simulink subsystem "global_to_local_waypoint_junho"  (R2022b)
settings: Solver=VariableStepAuto  StartTime=0.0  StopTime=10.0  RelTol=1e-3
libraries: CarMaker4SL x3
settings Model: Creator=USER  LastModifiedBy=USER

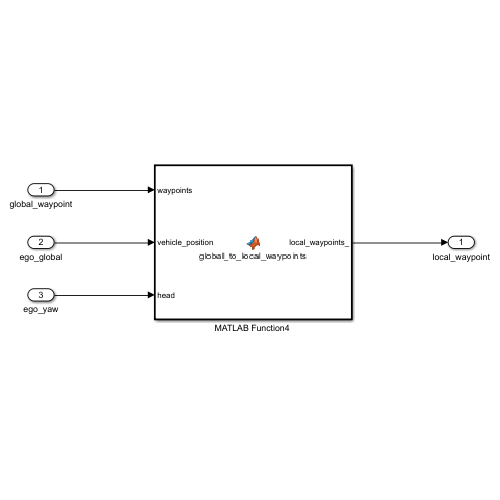
[thumbnail: Simulink's stored preview of the top-level diagram]
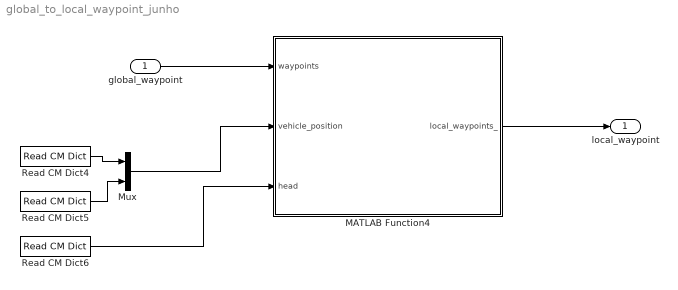
== system global_to_local_waypoint_junho ==
  global_waypoint : Inport
  "MATLAB Function4 " : MATLAB Function  TreatAsAtomicUnit=on
  Mux : Mux  Inputs=2
  Read CM Dict4 : CarMaker4SL/Read CM Dict  xname=Car.Fr1.tx  xsync=off  xstime=Inherited
  Read CM Dict5 : CarMaker4SL/Read CM Dict  xname=Car.Fr1.ty  xsync=off  xstime=Inherited
  Read CM Dict6 : CarMaker4SL/Read CM Dict  xname=Car.Fr1.rz  xsync=off  xstime=Inherited
  local_waypoint : Outport
  wires:
  "MATLAB Function4 "/1(local_waypoints_) -> local_waypoint/1
  global_waypoint/1 -> "MATLAB Function4 "/1(waypoints)
  Read CM Dict4/1 -> Mux/1
  Read CM Dict5/1 -> Mux/2
  Mux/1 -> "MATLAB Function4 "/2(vehicle_position)
  Read CM Dict6/1 -> "MATLAB Function4 "/3(head)

== matlab function global_to_local_waypoint_junho/MATLAB Function4  ==
  settings: updateMethod=DISCRETE  sampleTime=0.05
  data: waypoints input; local_waypoints_ output; vehicle_position input; head input
function local_waypoints_ = global_to_local_waypoints(waypoints, vehicle_position, head)
    num_waypoints = size(waypoints, 1);
    local_waypoints_ = zeros(num_waypoints, 2);

    % 헤딩 각에 대한 코사인 및 사인 계산
    cos_theta = cos(head);
    sin_theta = sin(head);

    for i = 1:num_waypoints
        % 글로벌 좌표에서 차량 위치를 빼서 상대적 위치 계산
        X_diff = waypoints(i, 1) - vehicle_position(1);
        Y_diff = waypoints(i, 2) - vehicle_position(2);
        
        % 2D 회전 변환을 통해 로컬 좌표로 변환
        local_waypoints_(i, 1) = X_diff * cos_theta + Y_diff * sin_theta;
        local_waypoints_(i, 2) = -X_diff * sin_theta + Y_diff * cos_theta;
    end
   
end
